simulink library "AEMS_Standard_Library"  (R2016b)
settings: Solver=ode45  StartTime=0.0  StopTime=10.0  RelTol=1e-3
undefined symbols (not defined in the file or in its folder): BkPY, carto, Cbx_extegr, Cbx_lpegrsys, Cbx_portegr, Cnx_bnk_nr_conf, Cnx_cyl_nr_conf, ConfigManagement, configuration_management, Cxx_dcm_io_tmr_end_xxxx, Cxx_dcm_rt_tmr_end, Cxx_DID_xxxx_IO_max, Cxx_DID_xxxx_IO_min, Cxx_egrhsofs, Cxx_vmaniegi, DEM_DEBOUNCE_FREEZE, DEM_DTR_CTL_INVISIBLE, DEM_DTR_CTL_NORMAL, Dem_DtrId2_XXX, Dem_DtrId3_XXX, Dem_DtrId4_XXX, Dem_DtrId5_XXX, Dem_DtrId6_XXX, Dem_DtrId7_XXX, Dem_DtrId8_XXX, Dem_DtrId9_XXX, Dem_DtrId_XXX, Dem_EnableConditionId2_XXX, Dem_EnableConditionId3_XXX, Dem_EnableConditionId4_XXX, Dem_EnableConditionId5_XXX, Dem_EnableConditionId6_XXX, Dem_EnableConditionId7_XXX, Dem_EnableConditionId8_XXX, Dem_EnableConditionId_XXX, Dem_EventId, Dem_EventId2_XXX, Dem_EventId3_XXX, Dem_EventId4_XXX, Dem_EventId5_XXX, Dem_EventId6_XXX, Dem_EventId7_XXX, Dem_EventId8_XXX, Dem_EventId9_XXX, Dem_EventId_Device_Faulttype, Dem_EventId_XXX, DEM_IUMPR_GENERAL_DENOMINATOR, DEM_OPCYC_IGNITION, Dem_RatioId2_XXX, Dem_RatioId3_XXX, Dem_RatioId4_XXX, Dem_RatioId5_XXX, Dem_RatioId6_XXX, Dem_RatioId7_XXX, Dem_RatioId8_XXX, Dem_RatioId_XXX, Dem_StorageConditionId2_XXX, Dem_StorageConditionId3_XXX, Dem_StorageConditionId4_XXX, Dem_StorageConditionId5_XXX ... (+65)
libraries: AEMS_Standard_Library x477, simulink x2
(part 37 of 39)

== system AEMS_Standard_Library/SPECIFIC/AEMS_AIR_BALANCE/MWI_Mani_Charge_Mass_Air_EGR/MWI_egrmani_pm_cal ==
  qcylegr_pudt : Inport  Interpolate=off
  fair_egrv : Inport  Port=2  Interpolate=off
  qegrve : Inport  Port=3  Interpolate=off
  egrmani_cal_ok : EnablePort
      settings: AttributesFormatString=<states=%<StatesWhenEnabling>>
  Product4 : Product  Inputs=*/  SaturateOnIntegerOverflow=on  RndMeth=Zero  InputSameDT=on
  Saturation1 : Saturate  UpperLimit=100  LowerLimit=0
      settings: AttributesFormatString=<limits=%<UpperLimit>/%<LowerLimit>>
  Sum : Sum  Inputs=+-  SaturateOnIntegerOverflow=on  InputSameDT=on
  Sum1 : Sum  SaturateOnIntegerOverflow=on  InputSameDT=on
  Switch : Switch  Criteria=u2 ~= 0  SaturateOnIntegerOverflow=on  InputSameDT=on
      settings: AttributesFormatString=Criteria=%<Criteria>
  Unit Delay3 : UnitDelay  SampleTime=-1
      settings: AttributesFormatString=<initial=%<InitialCondition>>
  g_per_s_to_g_per_freq : Constant  Value=500  OutDataTypeStr=single
  g_per_s_to_g_per_frq : Constant  Value=0  OutDataTypeStr=single
  egrmani : Outport  InitialOutput=0
      settings: AttributesFormatString=<initial=%<InitialOutput>>\n<whendisabled=%<OutputWhenDisabled>>
  wires:
  Product4/1 -> Sum1/2
  Unit Delay3/1 -> Sum1/1
  g_per_s_to_g_per_freq/1 -> Product4/2
  Saturation1/1 -> Unit Delay3/1, egrmani/1  "egrmani"
  Sum1/1 -> Saturation1/1
  Sum/1 -> Product4/1
  qcylegr_pudt/1 -> Sum/2
  qegrve/1 -> Switch/3
  g_per_s_to_g_per_frq/1 -> Switch/1
  fair_egrv/1 -> Switch/2
  Switch/1 -> Sum/1

== system AEMS_Standard_Library/SPECIFIC/AEMS_AIR_BALANCE/MWI_Mani_Charge_Mass_Air_EGR/MWI_mamani_pm_cal ==
  egrmani : Inport  Interpolate=off
  qegrth : Inport  Port=2  Interpolate=off
  fqselgo : Inport  Port=3  Interpolate=off
  pargeqd : Inport  Port=4  Interpolate=off
  tanmnp : Inport  Port=5  Interpolate=off
  ppamb : Inport  Port=6  Interpolate=off
  qtrm : Inport  Port=7  Interpolate=off
  qcyl_pudt : Inport  Port=8  Interpolate=off
  qcylall_pudt : Inport  Port=9  Interpolate=off
  fafmlmsta : Inport  Port=10  Interpolate=off
  vmani : Inport  Port=11  Interpolate=off
  qegrve : Inport  Port=12  Interpolate=off
  fair_egrv : Inport  Port=13  Interpolate=off
  Constant : Constant  Value=0  OutDataTypeStr=single
  Constant1 : Constant  Value=Cbx_lpegrsys
  Constant2 : Constant  Value=100  OutDataTypeStr=single
  MinMax : MinMax  Function=max  Inputs=2  SaturateOnIntegerOverflow=on  InputSameDT=on
  MinMax1 : MinMax  Inputs=2  SaturateOnIntegerOverflow=on  InputSameDT=on
  MinMax2 : MinMax  Function=max  Inputs=2  SaturateOnIntegerOverflow=on  InputSameDT=on
  Product : Product  Inputs=*/  SaturateOnIntegerOverflow=on  RndMeth=Zero  InputSameDT=on
  Product1 : Product  SaturateOnIntegerOverflow=on  RndMeth=Zero  InputSameDT=on
  Product2 : Product  SaturateOnIntegerOverflow=on  RndMeth=Zero  InputSameDT=on
  Product3 : Product  Inputs=*/  SaturateOnIntegerOverflow=on  RndMeth=Zero  InputSameDT=on
  Sum1 : Sum  Inputs=+-  SaturateOnIntegerOverflow=on  InputSameDT=on
  Sum{2..3,5..6} (4 alike) : Sum  SaturateOnIntegerOverflow=on  InputSameDT=on
  Sum4 : Sum  Inputs=+++  SaturateOnIntegerOverflow=on  InputSameDT=on
  Sum7 : Sum  Inputs=+-  SaturateOnIntegerOverflow=on  InputSameDT=on
  Switch{,1..3} (4 alike) : Switch  Criteria=u2 ~= 0  SaturateOnIntegerOverflow=on  InputSameDT=on
      settings: AttributesFormatString=Criteria=%<Criteria>
  Unit Delay1 : UnitDelay  SampleTime=-1
      settings: AttributesFormatString=<initial=%<InitialCondition>>
  constant : Constant  Value=0.00028704  OutDataTypeStr=single
  constant1 : Constant  Value=273  OutDataTypeStr=single
  constant2 : Constant  Value=0.00028704  OutDataTypeStr=single
  g/s_to_g/2ms1 : Constant  Value=500  OutDataTypeStr=single
  g/s_to_g/2ms2 : Constant  Value=0  OutDataTypeStr=single
  mVMANI1 : Constant  Value=Cxx_vmaniegi
  mamani : Outport
  airmani : Outport  Port=2
  wires:
  vmani/1 -> Sum5/2
  MinMax/1 -> Switch/3  "airmani"
  Switch2/1 -> MinMax1/1
  Sum2/1 -> MinMax1/2
  Constant/1 -> MinMax/2
  MinMax1/1 -> MinMax/1
  Constant2/1 -> Switch2/3
  fafmlmsta/1 -> Switch2/2
  pargeqd/1 -> Sum4/2
  qegrth/1 -> Sum7/2
  qcylall_pudt/1 -> Sum7/1
  Sum7/1 -> Switch1/1
  qcyl_pudt/1 -> Switch1/3
  Constant1/1 -> Switch1/2
  Switch1/1 -> Sum1/2
  Sum1/1 -> Product3/1
  constant2/1 -> MinMax2/1
  Product2/1 -> MinMax2/2
  MinMax2/1 -> Product/2
  egrmani/1 -> Sum6/2
  Sum6/1 -> mamani/1  "mamani"
  fqselgo/1 -> Switch/2
  Sum5/1 -> Product1/1
  mVMANI1/1 -> Sum5/1
  Switch/1 -> Sum6/1, Unit Delay1/1, airmani/1  "airmani"
  ppamb/1 -> Product1/2
  Product/1 -> Switch2/1, Switch/1  "mamani_ini"
  constant1/1 -> Sum3/2
  Sum3/1 -> Product2/2
  tanmnp/1 -> Sum3/1
  constant/1 -> Product2/1
  Product1/1 -> Product/1
  g/s_to_g/2ms1/1 -> Product3/2
  Product3/1 -> Sum2/1
  qtrm/1 -> Sum4/1
  Unit Delay1/1 -> Sum2/2
  Switch3/1 -> Sum4/3
  qegrve/1 -> Switch3/1
  g/s_to_g/2ms2/1 -> Switch3/3
  Sum4/1 -> Sum1/1
  fair_egrv/1 -> Switch3/2

== system AEMS_Standard_Library/SPECIFIC/AEMS_AS_PADE/A_pade_model/A_filter_pade ==
  Vxx_in_fil : Inport
  Vxx_dly_t : Inport  Port=2
  Vbx_dly_init_ena : Inport  Port=3
  A_filter_1 : Subsystem
  B_filter_2 : Subsystem
  C_filter_3 : Subsystem
  Vxx_in_dly : Outport
  wires:
  Vxx_dly_t/1 -> A_filter_1/1(Vxx_dly_t), C_filter_3/1(Vxx_dly_t), B_filter_2/1(Vxx_dly_t)
  Vbx_dly_init_ena/1 -> C_filter_3/3(Vbx_dly_init_ena), B_filter_2/3(Vbx_dly_init_ena), A_filter_1/3(Vbx_dly_init_ena)
  C_filter_3/1(Vxx_in_dly) -> Vxx_in_dly/1
  B_filter_2/1(Vxx_dly_2) -> C_filter_3/2(Vxx_dly_2)
  Vxx_in_fil/1 -> C_filter_3/4(Vxx_in_fil), B_filter_2/4(Vxx_in_fil), A_filter_1/2(Vxx_in_fil)
  A_filter_1/1(Vxx_dly_1) -> B_filter_2/2(Vxx_dly_1)

== system AEMS_Standard_Library/SPECIFIC/AEMS_AT_EHR/A_Enabled_Calculation/A_Calcul_for_all_bricks ==
  Vxx_ehr_cnvt_fac : Inport
  Vxx_ehr_ext_exch_ar : Inport  Port=2
  Vxx_ehr_samp_t : Inport  Port=3
  Product1 : Product  OutDataTypeStr=Inherit: Inherit via back propagation  RndMeth=Zero
  Product5 : Product  OutDataTypeStr=Inherit: Inherit via back propagation  RndMeth=Zero
  Vxx_ehr_ext_cnvt_entr : Outport
  wires:
  Product1/1 -> Vxx_ehr_ext_cnvt_entr/1
  Product5/1 -> Product1/1
  Vxx_ehr_samp_t/1 -> Product1/2
  Vxx_ehr_ext_exch_ar/1 -> Product5/2
  Vxx_ehr_cnvt_fac/1 -> Product5/1

== system AEMS_Standard_Library/SPECIFIC/AEMS_AT_EHR/A_Enabled_Calculation/B_Temp_calculation_in_brick ==
  Vxx_ehr_ext_cnvt_entr : Inport
  Vxx_ehr_samp_t : Inport  Port=2
  Vxx_ehr_sel_tenv : Inport  Port=3
  Vxx_ehr_spc_ex_gas_temp_cpy : Inport  Port=4
  Vxx_ehr_spc_cata_temp_cpy : Inport  Port=5
  Vxx_ehr_sys_egaf : Inport  Port=6
  Vxx_ehr_exo_pow : Inport  Port=7
  Vxx_ehr_wht : Inport  Port=8
  Vxx_ehr_utp : Inport  Port=9
  Vxx_ehr_cata_temp_dly : Inport  Port=10
  A_Entropy_calculation : Subsystem
  B_Temp_fluctuation_calculation : Subsystem
  C_Temp_and_power_calculation : Subsystem
  Saturation{,1..3} (4 alike) : Saturate  UpperLimit=1240  LowerLimit=0  RndMeth=Zero
      settings: AttributesFormatString=<limits=%<UpperLimit>/%<LowerLimit>>
  Saturation7 : Saturate  UpperLimit=32767  LowerLimit=-32767  RndMeth=Zero
      settings: AttributesFormatString=<limits=%<UpperLimit>/%<LowerLimit>>
  Vxx_ehr_dtp : Outport
  Vxx_ehr_ext_pow_loss : Outport  Port=2
  Vxx_ehr_wht_entr : Outport  Port=3
  Vxx_ehr_ex_gas_entr : Outport  Port=4
  Vxx_ehr_exo_temp_flu : Outport  Port=5
  Vxx_ehr_wht_temp_flu : Outport  Port=6
  Vxx_ehr_ex_gas_temp_flu : Outport  Port=7
  Vxx_ehr_ext_cnvt_temp_flu : Outport  Port=8
  wires:
  Saturation3/1 -> Vxx_ehr_ext_cnvt_temp_flu/1, C_Temp_and_power_calculation/4(Vxx_ehr_ext_cnvt_temp_flu)
  Saturation2/1 -> C_Temp_and_power_calculation/3(Vxx_ehr_ex_gas_temp_flu), Vxx_ehr_ex_gas_temp_flu/1
  Saturation1/1 -> Vxx_ehr_wht_temp_flu/1, C_Temp_and_power_calculation/2(Vxx_ehr_wht_temp_flu)
  Saturation/1 -> Vxx_ehr_exo_temp_flu/1, C_Temp_and_power_calculation/1(Vxx_ehr_exo_temp_flu)
  Saturation7/1 -> Vxx_ehr_ext_pow_loss/1
  C_Temp_and_power_calculation/1(Vxx_ehr_ext_pow_loss) -> Saturation7/1
  B_Temp_fluctuation_calculation/4(Vxx_ehr_ext_cnvt_temp_flu) -> Saturation3/1
  B_Temp_fluctuation_calculation/3(Vxx_ehr_ex_gas_temp_flu) -> Saturation2/1
  B_Temp_fluctuation_calculation/2(Vxx_ehr_wht_temp_flu) -> Saturation1/1
  B_Temp_fluctuation_calculation/1(Vxx_ehr_exo_temp_flu) -> Saturation/1
  A_Entropy_calculation/6(Vxx_ehr_ext_cnvt_entr_rat) -> B_Temp_fluctuation_calculation/4(Vxx_ehr_ext_cnvt_entr_rat)
  A_Entropy_calculation/5(Vxx_ehr_ex_gas_entr_rat) -> B_Temp_fluctuation_calculation/3(Vxx_ehr_ex_gas_entr_rat)
  C_Temp_and_power_calculation/2(Vxx_ehr_dtp) -> Vxx_ehr_dtp/1
  A_Entropy_calculation/4(Vxx_ehr_wht_entr_rat) -> B_Temp_fluctuation_calculation/2(Vxx_ehr_wht_entr_rat)
  A_Entropy_calculation/3(Vxx_ehr_ex_gas_entr) -> Vxx_ehr_ex_gas_entr/1
  A_Entropy_calculation/1(Vxx_ehr_entr_tot) -> B_Temp_fluctuation_calculation/1(Vxx_ehr_entr_tot)
  A_Entropy_calculation/2(Vxx_ehr_wht_entr) -> Vxx_ehr_wht_entr/1
  Vxx_ehr_wht/1 -> A_Entropy_calculation/4(Vxx_ehr_wht)
  Vxx_ehr_cata_temp_dly/1 -> B_Temp_fluctuation_calculation/8(Vxx_ehr_cata_temp_dly)
  Vxx_ehr_sys_egaf/1 -> A_Entropy_calculation/2(Vxx_ehr_sys_egaf)
  Vxx_ehr_exo_pow/1 -> B_Temp_fluctuation_calculation/6(Vxx_ehr_exo_pow)
  Vxx_ehr_spc_cata_temp_cpy/1 -> A_Entropy_calculation/1(Vxx_ehr_spc_cata_temp_cpy)
  Vxx_ehr_spc_ex_gas_temp_cpy/1 -> A_Entropy_calculation/3(Vxx_ehr_spc_ex_gas_temp_cpy)
  Vxx_ehr_ext_cnvt_entr/1 -> A_Entropy_calculation/5(Vxx_ehr_ext_cnvt_entr), C_Temp_and_power_calculation/7(Vxx_ehr_ext_cnvt_entr)
  Vxx_ehr_utp/1 -> B_Temp_fluctuation_calculation/7(Vxx_ehr_utp)
  Vxx_ehr_samp_t/1 -> A_Entropy_calculation/6(Vxx_ehr_samp_t), B_Temp_fluctuation_calculation/5(Vxx_ehr_samp_t), C_Temp_and_power_calculation/6(Vxx_ehr_samp_t)
  Vxx_ehr_sel_tenv/1 -> B_Temp_fluctuation_calculation/9(Vxx_ehr_sel_tenv), C_Temp_and_power_calculation/5(Vxx_ehr_sel_tenv)

== system AEMS_Standard_Library/SPECIFIC/AEMS_AT_TUBE/A_Thermal_Calculation/A_Thermal_Convection_Terms_Tube ==
  Vxx_tub_itl_cnvt_fac : Inport
  Vxx_tub_itl_ar : Inport  Port=2
  Vxx_tub_ext_cnvt_fac : Inport  Port=3
  Vxx_tub_ext_ar : Inport  Port=4
  hextSext : Product  Inputs=**  OutDataTypeStr=Inherit: Inherit via back propagation  RndMeth=Zero
  hextSext1 : Product  Inputs=**  OutDataTypeStr=Inherit: Inherit via back propagation  RndMeth=Zero
  Vxx_tub_ext_ar_cnvt_fac : Outport
  Vxx_tub_itl_ar_cnvt_fac : Outport  Port=2
  wires:
  Vxx_tub_itl_ar/1 -> hextSext1/2
  Vxx_tub_itl_cnvt_fac/1 -> hextSext1/1
  Vxx_tub_ext_ar/1 -> hextSext/2
  Vxx_tub_ext_cnvt_fac/1 -> hextSext/1
  hextSext1/1 -> Vxx_tub_itl_ar_cnvt_fac/1
  hextSext/1 -> Vxx_tub_ext_ar_cnvt_fac/1

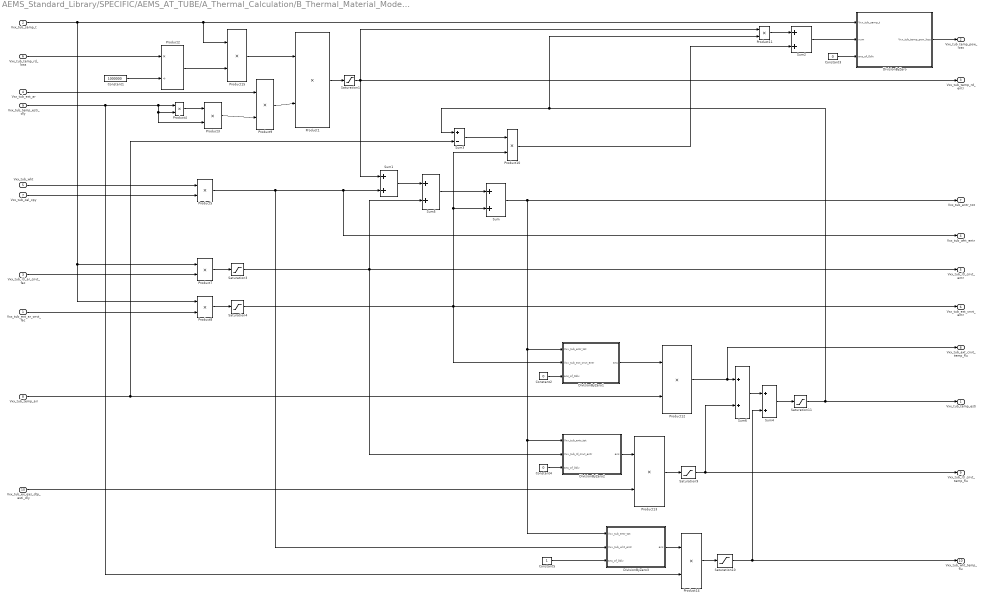
== system AEMS_Standard_Library/SPECIFIC/AEMS_AT_TUBE/A_Thermal_Calculation/B_Thermal_Material_Model_Tube ==
  Vxx_tub_ext_ar_cnvt_fac : Inport
  Vxx_tub_samp_t : Inport  Port=2
  Vxx_tub_itl_ar_cnvt_fac : Inport  Port=3
  Vxx_tub_ext_ar : Inport  Port=4
  Vxx_tub_wht : Inport  Port=5
  Vxx_tub_temp_rd_loss : Inport  Port=6
  Vxx_tub_cal_cpy : Inport  Port=7
  Vxx_tub_temp_air : Inport  Port=8
  Vxx_tub_temp_esti_dly : Inport  Port=9
  Vxx_tub_ex_gas_dtp_esti_dly : Inport  Port=10
  Constant1 : Constant  Value=1000000  OutDataTypeStr=Inherit: Inherit via back propagation
  Constant2 : Constant  Value=0  OutDataTypeStr=Inherit: Inherit via back propagation
  Constant3 : Constant  Value=0  OutDataTypeStr=Inherit: Inherit via back propagation
  Constant4 : Constant  Value=0  OutDataTypeStr=Inherit: Inherit via back propagation
  Constant5 : Constant  OutDataTypeStr=Inherit: Inherit via back propagation
  DivisionByZero : Subsystem
  DivisionByZero1 : Subsystem
  DivisionByZero2 : Subsystem
  DivisionByZero3 : Subsystem
  Product{1,3..4,9,15} (5 alike) : Product  OutDataTypeStr=Inherit: Inherit via back propagation  RndMeth=Zero
  Product{5,7..8,10..14} (8 alike) : Product  Inputs=**  OutDataTypeStr=Inherit: Inherit via back propagation  RndMeth=Zero
  Product2 : Product  Inputs=*/  OutDataTypeStr=Inherit: Inherit via back propagation  RndMeth=Zero
  Saturation1 : Saturate  UpperLimit=6.5535  LowerLimit=0  RndMeth=Zero
      settings: AttributesFormatString=<limits=%<UpperLimit>/%<LowerLimit>>
  Saturation10 : Saturate  UpperLimit=1240  LowerLimit=0  RndMeth=Zero
      settings: AttributesFormatString=<limits=%<UpperLimit>/%<LowerLimit>>
  Saturation11 : Saturate  UpperLimit=1473  LowerLimit=233  RndMeth=Zero
      settings: AttributesFormatString=<limits=%<UpperLimit>/%<LowerLimit>>
  Saturation3 : Saturate  UpperLimit=1310.6  LowerLimit=0  RndMeth=Zero
      settings: AttributesFormatString=<limits=%<UpperLimit>/%<LowerLimit>>
  Saturation4 : Saturate  UpperLimit=6.5535  LowerLimit=0  RndMeth=Zero
      settings: AttributesFormatString=<limits=%<UpperLimit>/%<LowerLimit>>
  Saturation9 : Saturate  UpperLimit=1240  LowerLimit=0  RndMeth=Zero
      settings: AttributesFormatString=<limits=%<UpperLimit>/%<LowerLimit>>
  Sum{,1..2,4..5} (5 alike) : Sum  Inputs=2  OutDataTypeStr=Inherit: Inherit via back propagation  RndMeth=Zero  InputSameDT=on
  Sum3 : Sum  Inputs=+-  OutDataTypeStr=Inherit: Inherit via back propagation  RndMeth=Zero  InputSameDT=on
  Sum6 : Sum  OutDataTypeStr=Inherit: Inherit via back propagation  RndMeth=Zero  InputSameDT=on
  Vxx_tub_temp_esti : Outport
  Vxx_tub_temp_pow_loss : Outport  Port=2
  Vxx_tub_temp_rd_entr : Outport  Port=3
  Vxx_tub_wht_entr : Outport  Port=4
  Vxx_tub_itl_cnvt_entr : Outport  Port=5
  Vxx_tub_ext_cnvt_entr : Outport  Port=6
  Vxx_tub_entr_tot : Outport  Port=7
  Vxx_tub_ext_cnvt_temp_flu : Outport  Port=8
  Vxx_tub_itl_cnvt_temp_flu : Outport  Port=9
  Vxx_tub_wht_temp_flu : Outport  Port=10
  wires:
  Saturation11/1 -> Vxx_tub_temp_esti/1, Product11/2, Sum3/1
  DivisionByZero/1(Vxx_tub_temp_pow_loss) -> Vxx_tub_temp_pow_loss/1
  Constant3/1 -> DivisionByZero/3(ans_of_0div)
  Sum2/1 -> DivisionByZero/2(num)
  Saturation9/1 -> Sum6/2, Vxx_tub_itl_cnvt_temp_flu/1
  Saturation10/1 -> Sum4/2, Vxx_tub_wht_temp_flu/1
  Saturation4/1 -> Vxx_tub_ext_cnvt_entr/1, Product10/2, Sum/2, DivisionByZero1/2(Vxx_tub_ext_cnvt_entr)
  Saturation3/1 -> DivisionByZero2/2(Vxx_tub_itl_cnvt_entr), Sum5/2, Vxx_tub_itl_cnvt_entr/1
  Saturation1/1 -> Sum1/1, Vxx_tub_temp_rd_entr/1, Product11/1
  Product9/1 -> Product1/2
  Product15/1 -> Product1/1
  Vxx_tub_ext_ar/1 -> Product9/1
  Product3/1 -> Product9/2
  Constant5/1 -> DivisionByZero3/3(ans_of_0div)
  Constant4/1 -> DivisionByZero2/3(ans_of_0div)
  Constant2/1 -> DivisionByZero1/3(ans_of_0div)
  Vxx_tub_temp_esti_dly/1 -> Product3/2, Product4/2, Product4/1, Product14/2
  Sum3/1 -> Product10/1
  Product10/1 -> Sum2/2
  Product11/1 -> Sum2/1
  Vxx_tub_temp_air/1 -> Sum3/2, Product12/2
  Vxx_tub_itl_ar_cnvt_fac/1 -> Product7/2
  Constant1/1 -> Product2/2
  Vxx_tub_temp_rd_loss/1 -> Product2/1
  Vxx_tub_cal_cpy/1 -> Product5/2
  Vxx_tub_wht/1 -> Product5/1
  Vxx_tub_ext_ar_cnvt_fac/1 -> Product8/2
  Product8/1 -> Saturation4/1
  DivisionByZero1/1(ans) -> Product12/1
  Product12/1 -> Sum6/1, Vxx_tub_ext_cnvt_temp_flu/1
  Product7/1 -> Saturation3/1
  Product13/1 -> Saturation9/1
  Product1/1 -> Saturation1/1
  Product5/1 -> DivisionByZero3/2(Vxx_tub_wht_entr), Vxx_tub_wht_entr/1, Sum1/2
  DivisionByZero3/1(ans) -> Product14/1
  Product14/1 -> Saturation10/1
  Sum4/1 -> Saturation11/1
  DivisionByZero2/1(ans) -> Product13/1
  Vxx_tub_ex_gas_dtp_esti_dly/1 -> Product13/2
  Product4/1 -> Product3/1
  Sum/1 -> DivisionByZero1/1(Vxx_tub_entr_tot), DivisionByZero2/1(Vxx_tub_entr_tot), DivisionByZero3/1(Vxx_tub_entr_tot), Vxx_tub_entr_tot/1
  Sum1/1 -> Sum5/1
  Sum5/1 -> Sum/1
  Sum6/1 -> Sum4/1
  Vxx_tub_samp_t/1 -> Product8/1, Product7/1, Product15/1, DivisionByZero/1(Vxx_tub_samp_t)
  Product2/1 -> Product15/2

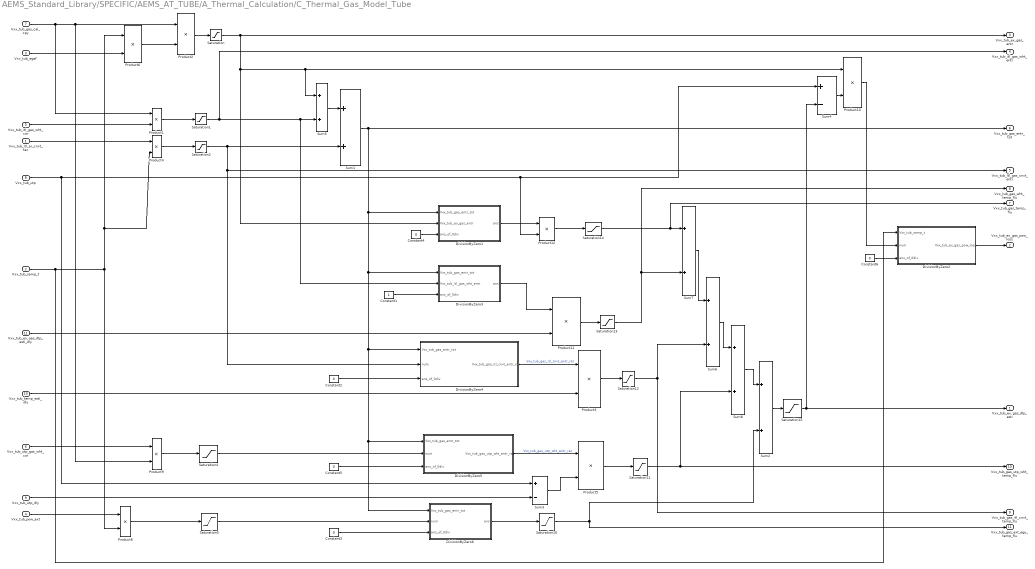
== system AEMS_Standard_Library/SPECIFIC/AEMS_AT_TUBE/A_Thermal_Calculation/C_Thermal_Gas_Model_Tube ==
  Vxx_tub_itl_ar_cnvt_fac : Inport
  Vxx_tub_samp_t : Inport  Port=2
  Vxx_tub_egaf : Inport  Port=3
  Vxx_tub_pow_ext : Inport  Port=4
  Vxx_tub_itl_gas_wht_cor : Inport  Port=5
  Vxx_tub_utp_gas_wht_cor : Inport  Port=6
  Vxx_tub_gas_cal_cpy : Inport  Port=7
  Vxx_tub_utp : Inport  Port=8
  Vxx_tub_utp_dly : Inport  Port=9
  Vxx_tub_temp_esti_dly : Inport  Port=10
  Vxx_tub_ex_gas_dtp_esti_dly : Inport  Port=11  PortDimensions=1
  Constant1 : Constant  OutDataTypeStr=Inherit: Inherit via back propagation
  Constant{2..6} (5 alike) : Constant  Value=0  OutDataTypeStr=Inherit: Inherit via back propagation
  DivisionByZero1 : Subsystem
  DivisionByZero2 : Subsystem
  DivisionByZero3 : Subsystem
  DivisionByZero4 : Subsystem
  DivisionByZero5 : Subsystem
  DivisionByZero6 : Subsystem
  Product{1..6,8..12} (11 alike) : Product  OutDataTypeStr=Inherit: Inherit via back propagation  RndMeth=Zero
  Saturation : Saturate  UpperLimit=65.535  LowerLimit=0  RndMeth=Zero
      settings: AttributesFormatString=<limits=%<UpperLimit>/%<LowerLimit>>
  Saturation1 : Saturate  UpperLimit=6553.5  LowerLimit=0  RndMeth=Zero
      settings: AttributesFormatString=<limits=%<UpperLimit>/%<LowerLimit>>
  Saturation10 : Saturate  UpperLimit=620  LowerLimit=-620  RndMeth=Zero
      settings: AttributesFormatString=<limits=%<UpperLimit>/%<LowerLimit>>
  Saturation11 : Saturate  UpperLimit=620  LowerLimit=-620  RndMeth=Zero
      settings: AttributesFormatString=<limits=%<UpperLimit>/%<LowerLimit>>
  Saturation12 : Saturate  UpperLimit=1240  LowerLimit=0  RndMeth=Zero
      settings: AttributesFormatString=<limits=%<UpperLimit>/%<LowerLimit>>
  Saturation13 : Saturate  UpperLimit=1240  LowerLimit=0  RndMeth=Zero
      settings: AttributesFormatString=<limits=%<UpperLimit>/%<LowerLimit>>
  Saturation14 : Saturate  UpperLimit=1240  LowerLimit=0  RndMeth=Zero
      settings: AttributesFormatString=<limits=%<UpperLimit>/%<LowerLimit>>
  Saturation15 : Saturate  UpperLimit=1473  LowerLimit=233  RndMeth=Zero
      settings: AttributesFormatString=<limits=%<UpperLimit>/%<LowerLimit>>
  Saturation2 : Saturate  UpperLimit=1310.6  LowerLimit=0  RndMeth=Zero
      settings: AttributesFormatString=<limits=%<UpperLimit>/%<LowerLimit>>
  Saturation4 : Saturate  UpperLimit=3276.7  LowerLimit=-3276.6  RndMeth=Zero
      settings: AttributesFormatString=<limits=%<UpperLimit>/%<LowerLimit>>
  Saturation5 : Saturate  UpperLimit=32767  LowerLimit=-32767  RndMeth=Zero
      settings: AttributesFormatString=<limits=%<UpperLimit>/%<LowerLimit>>
  Sum1 : Sum  Inputs=2  OutDataTypeStr=Inherit: Inherit via back propagation  RndMeth=Zero  InputSameDT=on
  Sum{2,6..8} (4 alike) : Sum  OutDataTypeStr=Inherit: Inherit via back propagation  RndMeth=Zero  InputSameDT=on
  Sum3 : Sum  Inputs=+-  OutDataTypeStr=Inherit: Inherit via back propagation  RndMeth=Zero  InputSameDT=on
  Sum4 : Sum  Inputs=+-  OutDataTypeStr=Inherit: Inherit via back propagation  RndMeth=Zero  InputSameDT=on
  Sum5 : Sum  Inputs=2  OutDataTypeStr=Inherit: Inherit via back propagation  RndMeth=Zero  InputSameDT=on
  Vxx_tub_ex_gas_dtp_esti : Outport
  Vxx_tub_ex_gas_pow_loss : Outport  Port=2
  Vxx_tub_ex_gas_entr : Outport  Port=3
  Vxx_tub_itl_gas_wht_entr : Outport  Port=4
  Vxx_tub_itl_gas_cnvt_entr : Outport  Port=5
  Vxx_tub_gas_entr_tot : Outport  Port=6
  Vxx_tub_gas_temp_flu : Outport  Port=7
  Vxx_tub_gas_wht_temp_flu : Outport  Port=8
  Vxx_tub_gas_itl_cnvt_temp_flu : Outport  Port=9
  Vxx_tub_gas_utp_wht_temp_flu : Outport  Port=10
  Vxx_tub_gas_ext_egy_temp_flu : Outport  Port=11
  wires:
  Sum1/1 -> DivisionByZero6/1(Vxx_tub_gas_entr_tot), DivisionByZero5/1(Vxx_tub_gas_entr_tot), DivisionByZero4/1(Vxx_tub_gas_entr_tot), DivisionByZero3/1(Vxx_tub_gas_entr_tot), DivisionByZero1/1(Vxx_tub_gas_entr_tot), Vxx_tub_gas_entr_tot/1
  Saturation4/1 -> DivisionByZero5/2(num)
  Saturation5/1 -> DivisionByZero6/2(num)
  Saturation14/1 -> Sum7/1, Vxx_tub_gas_temp_flu/1
  DivisionByZero2/1(Vxx_tub_ex_gas_pow_loss) -> Vxx_tub_ex_gas_pow_loss/1
  Product10/1 -> DivisionByZero2/2(num)
  Constant6/1 -> DivisionByZero2/3(ans_of_0div)
  Saturation15/1 -> Vxx_tub_ex_gas_dtp_esti/1, Sum4/2
  Saturation11/1 -> Sum8/2, Vxx_tub_gas_utp_wht_temp_flu/1
  Saturation12/1 -> Sum6/2, Vxx_tub_gas_itl_cnvt_temp_flu/1
  Saturation13/1 -> Sum7/2, Vxx_tub_gas_wht_temp_flu/1
  Saturation10/1 -> Sum2/2, Vxx_tub_gas_ext_egy_temp_flu/1
  Saturation2/1 -> DivisionByZero4/2(num), Vxx_tub_itl_gas_cnvt_entr/1, Sum1/2
  Saturation1/1 -> DivisionByZero3/2(Vxx_tub_itl_gas_wht_entr), Sum5/2, Vxx_tub_itl_gas_wht_entr/1
  Saturation/1 -> Vxx_tub_ex_gas_entr/1, DivisionByZero1/2(Vxx_tub_ex_gas_entr), Sum5/1, Product10/1
  Sum4/1 -> Product10/2
  Vxx_tub_utp_dly/1 -> Sum3/2
  Sum3/1 -> Product5/2
  Vxx_tub_pow_ext/1 -> Product8/1
  Vxx_tub_itl_ar_cnvt_fac/1 -> Product4/1
  Vxx_tub_temp_esti_dly/1 -> Product3/2
  Vxx_tub_ex_gas_dtp_esti_dly/1 -> Product11/2
  Constant5/1 -> DivisionByZero5/3(ans_of_0div)
  Constant4/1 -> DivisionByZero1/3(ans_of_0div)
  Constant3/1 -> DivisionByZero6/3(ans_of_0div)
  Constant2/1 -> DivisionByZero4/3(ans_of_0div)
  Constant1/1 -> DivisionByZero3/3(ans_of_0div)
  Vxx_tub_utp_gas_wht_cor/1 -> Product9/1
  Vxx_tub_itl_gas_wht_cor/1 -> Product1/2
  Vxx_tub_egaf/1 -> Product6/2
  Product2/1 -> Saturation/1
  Product8/1 -> Saturation5/1
  DivisionByZero1/1(ans) -> Product12/1
  DivisionByZero6/1(ans) -> Saturation10/1
  DivisionByZero4/1(Vxx_tub_gas_itl_cnvt_entr_rat) -> Product3/1  "Vxx_tub_gas_itl_cnvt_entr_rat"
  Product3/1 -> Saturation12/1
  Product12/1 -> Saturation14/1
  DivisionByZero5/1(Vxx_tub_gas_utp_wht_entr_rat) -> Product5/1  "Vxx_tub_gas_utp_wht_entr_rat"
  Product5/1 -> Saturation11/1
  DivisionByZero3/1(ans) -> Product11/1
  Product11/1 -> Saturation13/1
  Product4/1 -> Saturation2/1
  Product1/1 -> Saturation1/1
  Product9/1 -> Saturation4/1
  Sum2/1 -> Saturation15/1
  Sum5/1 -> Sum1/1
  Sum6/1 -> Sum8/1
  Sum7/1 -> Sum6/1
  Sum8/1 -> Sum2/1
  Vxx_tub_gas_cal_cpy/1 -> Product9/2, Product2/1, Product1/1
  Vxx_tub_utp/1 -> Sum4/1, Product12/2, Sum3/1
  Vxx_tub_samp_t/1 -> DivisionByZero2/1(Vxx_tub_samp_t), Product4/2, Product6/1, Product8/2
  Product6/1 -> Product2/2

== system AEMS_Standard_Library/SPECIFIC/AEMS_MULTIPORT_TIMESWITCH_CONFIG/slop_on/SR_FlipFlop ==
  S : Inport
  R : Inport  Port=2
  Constant3 : Constant  Value=true
  Constant5 : Constant  Value=false
  Logical_Operator : Logic  OutDataTypeStr=boolean
  Logical_Operator3 : Logic  Operator=NOT  OutDataTypeStr=boolean
  Switch1 : Switch  Criteria=u2 ~= 0  RndMeth=Zero  InputSameDT=on
      settings: AttributesFormatString=Criteria=%<Criteria>
  Switch2 : Switch  Criteria=u2 ~= 0  RndMeth=Zero  InputSameDT=on
      settings: AttributesFormatString=Criteria=%<Criteria>
  Switch3 : Switch  Criteria=u2 ~= 0  RndMeth=Zero  InputSameDT=on
      settings: AttributesFormatString=Criteria=%<Criteria>
  Unit_Delay : UnitDelay  InitialCondition=initial_condition  SampleTime=-1
      settings: AttributesFormatString=<initial=%<InitialCondition>>
  Q : Outport
  QNot : Outport  Port=2
  wires:
  Logical_Operator3/1 -> QNot/1
  Switch1/1 -> Q/1, Unit_Delay/1, Logical_Operator3/1
  Switch2/1 -> Switch1/3
  Switch3/1 -> Switch2/3
  Constant5/1 -> Switch3/1
  Constant3/1 -> Switch2/1
  Unit_Delay/1 -> Switch3/3, Switch1/1
  S/1 -> Logical_Operator/1, Switch2/2
  R/1 -> Logical_Operator/2, Switch3/2
  Logical_Operator/1 -> Switch1/2

== system AEMS_Standard_Library/SPECIFIC/AEMS_MULTIPORT_TIMESWITCH_CONFIG/transient_timer/DivisionByZero ==
  den : Inport
  num : Inport  Port=2
  ans_of_0div : Inport  Port=3
  Divide : Product  Inputs=*/  OutDataTypeStr=Inherit: Inherit via back propagation  RndMeth=Zero
  MinMax1 : MinMax  Function=max  Inputs=2  OutDataTypeStr=Inherit: Inherit via back propagation  RndMeth=Zero  InputSameDT=on
  RelationalOperator : RelationalOperator  Operator=~=  OutDataTypeStr=boolean  RndMeth=Nearest  InputSameDT=on
  Switch1 : Switch  Criteria=u2 ~= 0  RndMeth=Zero  SaturateOnIntegerOverflow=on  InputSameDT=on
      settings: AttributesFormatString=Criteria=%<Criteria>
  imm_zero : Constant  Value=0  OutDataTypeStr=Inherit: Inherit via back propagation
  imm_zero3 : Constant  Value=1.1920929e-07  OutDataTypeStr=Inherit: Inherit via back propagation
  ans : Outport
  wires:
  imm_zero3/1 -> MinMax1/2
  MinMax1/1 -> Divide/2
  den/1 -> MinMax1/1, RelationalOperator/1
  ans_of_0div/1 -> Switch1/3
  Divide/1 -> Switch1/1
  num/1 -> Divide/1
  Switch1/1 -> ans/1
  imm_zero/1 -> RelationalOperator/2
  RelationalOperator/1 -> Switch1/2

== system AEMS_Standard_Library/SPECIFIC/AEMS_MULTIPORT_TIMESWITCH_CONFIG/transient_timer/UnitDelayResettable ==
  u : Inport
  R : Inport  Port=2
  FixPt_Constant : Constant  DisableCoverage=on  Value=true
  FixPt_Logical_Operator : Logic  DisableCoverage=on  Operator=OR  OutDataTypeStr=boolean
  FixPt_Logical_Operator1 : Logic  DisableCoverage=on  Operator=NOT  OutDataTypeStr=boolean
  FixPt_Unit_Delay1 : UnitDelay  DisableCoverage=on  SampleTime=-1
      settings: AttributesFormatString=<initial=%<InitialCondition>>
  FixPt_Unit_Delay2 : UnitDelay  DisableCoverage=on  InitialCondition=false  SampleTime=-1
      settings: AttributesFormatString=<initial=%<InitialCondition>>
  Init : Switch  Criteria=u2 ~= 0  RndMeth=Zero  ZeroCross=off  InputSameDT=on
      settings: AttributesFormatString=Criteria=%<Criteria>
  Initial_Condition : Constant  DisableCoverage=on  Value=0  OutDataTypeStr=Inherit: Inherit via back propagation
  Reset : Switch  Criteria=u2 ~= 0  RndMeth=Zero  ZeroCross=off  InputSameDT=on
      settings: AttributesFormatString=Criteria=%<Criteria>
  y : Outport
  wires:
  u/1 -> Reset/3
  Initial_Condition/1 -> Reset/1, Init/1  "Initial_Value"
  R/1 -> Reset/2, FixPt_Logical_Operator/1
  FixPt_Logical_Operator/1 -> Init/2
  FixPt_Constant/1 -> FixPt_Unit_Delay2/1
  FixPt_Logical_Operator1/1 -> FixPt_Logical_Operator/2
  Reset/1 -> FixPt_Unit_Delay1/1  "Xnew"
  FixPt_Unit_Delay1/1 -> Init/3  "Xold"
  Init/1 -> y/1
  FixPt_Unit_Delay2/1 -> FixPt_Logical_Operator1/1

== system AEMS_Standard_Library/SPECIFIC/AEMS_SlopeSwitchExtern/Slope_On_Block/Error_Due_To_High_Slope_Test ==
  Signal_Change : Inport
  Output_Less_Than_Input : Inport  Port=2
  Output_Greater_Than_Input : Inport  Port=3
  Logical_Operator1 : Logic  Operator=OR  OutDataTypeStr=boolean
  Relational_Operator3 : RelationalOperator  Operator=~=  OutDataTypeStr=boolean  RndMeth=Nearest  InputSameDT=on
  Unit_Delay1 : UnitDelay  InitialCondition=false  SampleTime=-1
      settings: AttributesFormatString=<initial=%<InitialCondition>>
  Test_passed : Outport
  wires:
  Logical_Operator1/1 -> Test_passed/1
  Signal_Change/1 -> Logical_Operator1/1
  Output_Less_Than_Input/1 -> Unit_Delay1/1
  Output_Greater_Than_Input/1 -> Relational_Operator3/1
  Relational_Operator3/1 -> Logical_Operator1/2
  Unit_Delay1/1 -> Relational_Operator3/2

== system AEMS_Standard_Library/SPECIFIC/AEMS_SlopeSwitchExtern/Slope_On_Block/Output_Comparision ==
  Test_passed : Inport
  Input : Inport  Port=2
  Pos_Slope : Inport  Port=3
  Prev_Output : Inport  Port=4
  Neg_Slope : Inport  Port=5
  Logical_Operator : Logic  Operator=OR  OutDataTypeStr=boolean
  Logical_Operator2 : Logic  OutDataTypeStr=boolean
  Relational_Operator1 : RelationalOperator  Operator=>  OutDataTypeStr=boolean  RndMeth=Nearest  InputSameDT=on
  Relational_Operator2 : RelationalOperator  Operator=<  OutDataTypeStr=boolean  RndMeth=Nearest  InputSameDT=on
  Sum : Sum  OutDataTypeStr=Inherit: Inherit via back propagation  RndMeth=Zero  InputSameDT=on
  Sum1 : Sum  OutDataTypeStr=Inherit: Inherit via back propagation  RndMeth=Zero  InputSameDT=on
  Switch1 : Switch  Criteria=u2 ~= 0  RndMeth=Zero  SaturateOnIntegerOverflow=on  InputSameDT=on
      settings: AttributesFormatString=Criteria=%<Criteria>
  Switch2 : Switch  Criteria=u2 ~= 0  RndMeth=Zero  SaturateOnIntegerOverflow=on  InputSameDT=on
      settings: AttributesFormatString=Criteria=%<Criteria>
  Switch3 : Switch  Criteria=u2 ~= 0  RndMeth=Zero  SaturateOnIntegerOverflow=on  InputSameDT=on
      settings: AttributesFormatString=Criteria=%<Criteria>
  Output_Not_Equals_Input : Outport
  Output : Outport  Port=2
  Output_Less_Than_Input : Outport  Port=3
  Output_Greater_Than_Input : Outport  Port=4
  wires:
  Relational_Operator2/1 -> Output_Less_Than_Input/1, Logical_Operator/1, Switch2/2
  Input/1 -> Relational_Operator2/2, Relational_Operator1/2, Switch1/3, Switch3/3
  Switch2/1 -> Switch3/1
  Switch1/1 -> Switch2/3
  Sum/1 -> Relational_Operator1/1, Switch1/1
  Logical_Operator2/1 -> Output_Not_Equals_Input/1
  Logical_Operator/1 -> Logical_Operator2/2
  Switch3/1 -> Output/1
  Test_passed/1 -> Logical_Operator2/1, Switch3/2
  Relational_Operator1/1 -> Logical_Operator/2, Output_Greater_Than_Input/1, Switch1/2
  Sum1/1 -> Relational_Operator2/1, Switch2/1
  Pos_Slope/1 -> Sum1/1
  Prev_Output/1 -> Sum1/2, Sum/1
  Neg_Slope/1 -> Sum/2

== system AEMS_Standard_Library/COM/AEMS_FRAME_SUPERVISION/ecu_frm_monitoring/B_Status_Management/C_Status_building ==
  Mon_Authorize : Inport
  TimeSched_dt : Inport  Port=2
  JT1 : Inport  Port=3
  JT2 : Inport  Port=4
  Frame_Received : Inport  Port=5
  Status_PREV : Inport  Port=6
  AEMS_UNITDELAY_EXTERNALIC : AEMS_Standard_Library/DISCRETE/AEMS_UNITDELAY_EXTERNALIC  Tag=[LIB]
      settings: AttributesFormatString=%<MaskType>
  Constant2 : Constant  Value=-1  OutDataTypeStr=Inherit: Inherit via back propagation
  Constant4 : Constant  Value=0  OutDataTypeStr=Inherit: Inherit via back propagation
  Constant5 : Constant  Value=false
  DataTypeConversion2 : DataTypeConversion  RndMeth=Zero
  LogicalOperator1 : Logic  Operator=OR  OutDataTypeStr=boolean
  LogicalOperator2 : Logic  Inputs=3  OutDataTypeStr=boolean
  LogicalOperator4 : Logic  Operator=NOT  OutDataTypeStr=boolean
  LogicalOperator5 : Logic  OutDataTypeStr=boolean
  Nsx_abst : Constant  Value=Nnx_abst_stt
  Nsx_pres : Constant  Value=Nnx_pres_stt
  Nsx_vld_abst : Constant  Value=Nnx_vld_abst_stt
  Product : Product  OutDataTypeStr=Inherit: Inherit via back propagation  RndMeth=Zero
  RelationalOperator1 : RelationalOperator  OutDataTypeStr=boolean  RndMeth=Nearest  InputSameDT=on
  RelationalOperator2 : RelationalOperator  OutDataTypeStr=boolean  RndMeth=Nearest  InputSameDT=on
  RelationalOperator3 : RelationalOperator  OutDataTypeStr=boolean  RndMeth=Nearest  InputSameDT=on
  RelationalOperator4 : RelationalOperator  Operator=~=  OutDataTypeStr=boolean  RndMeth=Nearest  InputSameDT=on
  Sum1 : Sum  OutDataTypeStr=Inherit: Inherit via back propagation  RndMeth=Zero  InputSameDT=on
  Sum2 : Sum  Inputs=+-  OutDataTypeStr=Inherit: Inherit via back propagation  RndMeth=Zero  InputSameDT=on
  Switch{1..6} (6 alike) : Switch  Criteria=u2 ~= 0  RndMeth=Zero  InputSameDT=on
      settings: AttributesFormatString=Criteria=%<Criteria>
  UnitDelay2 : UnitDelay  InitialCondition=true  SampleTime=-1
      settings: AttributesFormatString=<initial=%<InitialCondition>>
  UnitDelay3 : UnitDelay  InitialCondition=true  SampleTime=-1
      settings: AttributesFormatString=<initial=%<InitialCondition>>
  Status : Outport
      settings: AttributesFormatString=%<SignalName>
  wires:
  Switch1/1 -> RelationalOperator2/1, RelationalOperator3/1, AEMS_UNITDELAY_EXTERNALIC/1
  Switch4/1 -> Switch6/3
  Sum2/1 -> RelationalOperator1/2
  AEMS_UNITDELAY_EXTERNALIC/1 -> RelationalOperator1/1, Sum1/2
  RelationalOperator1/1 -> Switch3/2
  Sum1/1 -> Switch3/3
  Constant4/1 -> Switch1/1
  Switch3/1 -> Switch1/3
  JT2/1 -> RelationalOperator2/2, Switch3/1, Sum2/1
  RelationalOperator2/1 -> LogicalOperator5/1
  JT1/1 -> RelationalOperator3/2
  Switch2/1 -> Switch4/3
  Nsx_pres/1 -> RelationalOperator4/2, Switch4/1
  Constant5/1 -> UnitDelay2/1
  Mon_Authorize/1 -> LogicalOperator2/2, UnitDelay3/1, LogicalOperator5/2
  LogicalOperator1/1 -> Switch1/2
  UnitDelay3/1 -> LogicalOperator4/1
  LogicalOperator4/1 -> LogicalOperator2/1
  LogicalOperator2/1 -> LogicalOperator1/1
  RelationalOperator4/1 -> LogicalOperator2/3
  DataTypeConversion2/1 -> Status/1
  TimeSched_dt/1 -> Product/1, Sum1/1, Sum2/2
  Constant2/1 -> Product/2
  Product/1 -> AEMS_UNITDELAY_EXTERNALIC/2
  Switch5/1 -> Switch2/3
  Switch6/1 -> DataTypeConversion2/1
  Status_PREV/1 -> Switch6/1, Switch5/3, RelationalOperator4/1
  Frame_Received/1 -> Switch4/2, LogicalOperator1/2
  LogicalOperator5/1 -> Switch2/2
  RelationalOperator3/1 -> Switch5/2
  UnitDelay2/1 -> Switch6/2
  Nsx_abst/1 -> Switch5/1
  Nsx_vld_abst/1 -> Switch2/1

== system AEMS_Standard_Library/MATH/AEMS_SORT/For_loop_1/For_loop_2/Comparison ==
  Vector : Inport
  Index_vector : Inport  Port=2
  Add : Sum
  Constant : Constant  OutDataTypeStr=int8
  Relational_Operator : RelationalOperator  Operator=>  OutDataTypeStr=boolean  RndMeth=Simplest  InputSameDT=on
  Selector : Selector  IndexMode=Zero-based  InputPortWidth=N  IndexOptions=Index vector (port)  Indices=[1 3]  OutputSizes=1
  Selector1 : Selector  IndexMode=Zero-based  InputPortWidth=N  IndexOptions=Index vector (port)  Indices=[1 3]  OutputSizes=1
  Relational_Operator_Boolean : Outport
  High_value_Out : Outport  Port=2
  Low_value_Out : Outport  Port=3
  Low_index_Out : Outport  Port=4
  wires:
  Vector/1 -> Selector/1, Selector1/1
  Index_vector/1 -> Add/1, Selector/2
  Constant/1 -> Add/2
  Selector1/1 -> Low_value_Out/1, Relational_Operator/2
  Add/1 -> Low_index_Out/1, Selector1/2
  Selector/1 -> High_value_Out/1, Relational_Operator/1
  Relational_Operator/1 -> Relational_Operator_Boolean/1

== system AEMS_Standard_Library/MATH/AEMS_SORT/For_loop_1/For_loop_2/Permutation_false ==
  Vector : Inport
  Action Port : ActionPort
  Non_permuted_vector : Outport
  wires:
  Vector/1 -> Non_permuted_vector/1

== system AEMS_Standard_Library/MATH/AEMS_SORT/For_loop_1/For_loop_2/Permutation_true ==
  High_value : Inport
  Low_value : Inport  Port=2
  Low_index : Inport  Port=3
  High_index : Inport  Port=4
  Vector : Inport  Port=5
  Action Port : ActionPort
  Assignment : Assignment  IndexMode=Zero-based  DiagnosticForDimensions=Warning  IndexOptions=Index vector (port)  Indices=1  OutputSizes=1
  Mux : Mux  Inputs=2
  Mux2 : Mux  Inputs=2
  Permuted_vector : Outport
  wires:
  Vector/1 -> Assignment/1
  Mux/1 -> Assignment/2
  Low_value/1 -> Mux/2
  Mux2/1 -> Assignment/3
  Assignment/1 -> Permuted_vector/1
  High_value/1 -> Mux/1
  Low_index/1 -> Mux2/1
  High_index/1 -> Mux2/2

== system AEMS_Standard_Library/MATH/AEMS_SORT/For_loop_1/For_loop_2/Unit_delay_vector ==
  Previous_vector : Inport
  Vector_to_sort : Inport  Port=2
  Index_vector : Inport  Port=3
  Constant1 : Constant  Value=0  OutDataTypeStr=int8
  Logical Operator : Logic  OutDataTypeStr=boolean
  RelationalOperator1 : RelationalOperator  Operator===  OutDataTypeStr=boolean  RndMeth=Nearest  InputSameDT=on
  Switch : Switch  Criteria=u2 ~= 0  RndMeth=Zero  SaturateOnIntegerOverflow=on
      settings: AttributesFormatString=Criteria=%<Criteria>
  UnitDelay1 : UnitDelay  InitialCondition=true  SampleTime=-1
      settings: AttributesFormatString=<initial=%<InitialCondition>>
  Vector_being_sorted : Outport
  wires:
  Logical Operator/1 -> Switch/2
  UnitDelay1/1 -> Logical Operator/2
  RelationalOperator1/1 -> Logical Operator/1, UnitDelay1/1
  Index_vector/1 -> RelationalOperator1/1
  Constant1/1 -> RelationalOperator1/2
  Previous_vector/1 -> Switch/3
  Switch/1 -> Vector_being_sorted/1
  Vector_to_sort/1 -> Switch/1

== system AEMS_Standard_Library/SPECIFIC/AEMS_AS_PADE/A_pade_model/A_filter_pade/A_filter_1 ==
  Vxx_dly_t : Inport
  Vxx_in_fil : Inport  Port=2
  Vbx_dly_init_ena : Inport  Port=3
  AEMS_LUT_1D : AEMS_Standard_Library/LOOKUP_TABLES/AEMS_LUT_1D  Tag=[LIB]  map_x=Cxb_lb_dly_t_para  map_z=Cxp_lb_b0_1
      settings: AttributesFormatString=%<MaskType>\nBkPX=%<map_x>\nLUT=%<map_z>
  AEMS_LUT_1D1 : AEMS_Standard_Library/LOOKUP_TABLES/AEMS_LUT_1D  Tag=[LIB]  map_x=Cxb_lb_dly_t_para  map_z=Cxp_lb_b1_1
      settings: AttributesFormatString=%<MaskType>\nBkPX=%<map_x>\nLUT=%<map_z>
  AEMS_LUT_1D2 : AEMS_Standard_Library/LOOKUP_TABLES/AEMS_LUT_1D  Tag=[LIB]  map_x=Cxb_lb_dly_t_para  map_z=Cxp_lb_a1_1
      settings: AttributesFormatString=%<MaskType>\nBkPX=%<map_x>\nLUT=%<map_z>
  AEMS_LUT_1D3 : AEMS_Standard_Library/LOOKUP_TABLES/AEMS_LUT_1D  Tag=[LIB]  map_x=Cxb_lb_dly_t_para  map_z=Cxp_lb_a2_1
      settings: AttributesFormatString=%<MaskType>\nBkPX=%<map_x>\nLUT=%<map_z>
  A_pade_2nd_order_filter_1 : Subsystem
  Constant1 : Constant  OutDataTypeStr=Inherit: Inherit via back propagation
  Saturation : Saturate  UpperLimit=2000  LowerLimit=0  RndMeth=Zero
      settings: AttributesFormatString=<limits=%<UpperLimit>/%<LowerLimit>>
  Sum1 : Sum  OutDataTypeStr=Inherit: Inherit via back propagation  RndMeth=Zero  InputSameDT=on
  Sum2 : Sum  OutDataTypeStr=Inherit: Inherit via back propagation  RndMeth=Zero  InputSameDT=on
  Sum3 : Sum  Inputs=+-  OutDataTypeStr=Inherit: Inherit via back propagation  RndMeth=Zero  InputSameDT=on
  Sum4 : Sum  Inputs=+-  OutDataTypeStr=Inherit: Inherit via back propagation  RndMeth=Zero  InputSameDT=on
  Vxx_dly_1 : Outport
  wires:
  AEMS_LUT_1D3/1 -> A_pade_2nd_order_filter_1/5(Vxx_a2_1), Sum2/2
  AEMS_LUT_1D2/1 -> A_pade_2nd_order_filter_1/4(Vxx_a1_1), Sum1/2
  AEMS_LUT_1D1/1 -> A_pade_2nd_order_filter_1/2(Vxx_b1_1), Sum3/2
  AEMS_LUT_1D/1 -> A_pade_2nd_order_filter_1/1(Vxx_b0_1), Sum4/2
  Vbx_dly_init_ena/1 -> A_pade_2nd_order_filter_1/7(Vbx_dly_init_ena)
  A_pade_2nd_order_filter_1/1(Vxx_dly_1) -> Saturation/1
  Vxx_in_fil/1 -> A_pade_2nd_order_filter_1/6(Vxx_in_fil)
  Vxx_dly_t/1 -> AEMS_LUT_1D/1, AEMS_LUT_1D1/1, AEMS_LUT_1D2/1, AEMS_LUT_1D3/1
  Sum4/1 -> A_pade_2nd_order_filter_1/3(Vxx_b2_1)
  Constant1/1 -> Sum1/1
  Sum1/1 -> Sum2/1
  Sum2/1 -> Sum3/1
  Sum3/1 -> Sum4/1
  Saturation/1 -> Vxx_dly_1/1

== system AEMS_Standard_Library/SPECIFIC/AEMS_AS_PADE/A_pade_model/A_filter_pade/B_filter_2 ==
  Vxx_dly_t : Inport
  Vxx_dly_1 : Inport  Port=2
  Vbx_dly_init_ena : Inport  Port=3
  Vxx_in_fil : Inport  Port=4
  AEMS_LUT_1D : AEMS_Standard_Library/LOOKUP_TABLES/AEMS_LUT_1D  Tag=[LIB]  map_x=Cxb_lb_dly_t_para  map_z=Cxp_lb_b0_2
      settings: AttributesFormatString=%<MaskType>\nBkPX=%<map_x>\nLUT=%<map_z>
  AEMS_LUT_1D1 : AEMS_Standard_Library/LOOKUP_TABLES/AEMS_LUT_1D  Tag=[LIB]  map_x=Cxb_lb_dly_t_para  map_z=Cxp_lb_b1_2
      settings: AttributesFormatString=%<MaskType>\nBkPX=%<map_x>\nLUT=%<map_z>
  AEMS_LUT_1D2 : AEMS_Standard_Library/LOOKUP_TABLES/AEMS_LUT_1D  Tag=[LIB]  map_x=Cxb_lb_dly_t_para  map_z=Cxp_lb_a1_2
      settings: AttributesFormatString=%<MaskType>\nBkPX=%<map_x>\nLUT=%<map_z>
  AEMS_LUT_1D3 : AEMS_Standard_Library/LOOKUP_TABLES/AEMS_LUT_1D  Tag=[LIB]  map_x=Cxb_lb_dly_t_para  map_z=Cxp_lb_a2_2
      settings: AttributesFormatString=%<MaskType>\nBkPX=%<map_x>\nLUT=%<map_z>
  A_pade_2nd_order_filter_2 : Subsystem
  Constant1 : Constant  OutDataTypeStr=Inherit: Inherit via back propagation
  Saturation : Saturate  UpperLimit=2000  LowerLimit=0  RndMeth=Zero
      settings: AttributesFormatString=<limits=%<UpperLimit>/%<LowerLimit>>
  Sum1 : Sum  OutDataTypeStr=Inherit: Inherit via back propagation  RndMeth=Zero  InputSameDT=on
  Sum2 : Sum  OutDataTypeStr=Inherit: Inherit via back propagation  RndMeth=Zero  InputSameDT=on
  Sum3 : Sum  Inputs=+-  OutDataTypeStr=Inherit: Inherit via back propagation  RndMeth=Zero  InputSameDT=on
  Sum4 : Sum  Inputs=+-  OutDataTypeStr=Inherit: Inherit via back propagation  RndMeth=Zero  InputSameDT=on
  Vxx_dly_2 : Outport
  wires:
  Vxx_in_fil/1 -> A_pade_2nd_order_filter_2/8(Vxx_in_fil)
  Vbx_dly_init_ena/1 -> A_pade_2nd_order_filter_2/7(Vbx_dly_init_ena)
  Vxx_dly_t/1 -> AEMS_LUT_1D/1, AEMS_LUT_1D1/1, AEMS_LUT_1D2/1, AEMS_LUT_1D3/1
  Vxx_dly_1/1 -> A_pade_2nd_order_filter_2/6(Vxx_dly_1)
  A_pade_2nd_order_filter_2/1(Vxx_dly_2) -> Saturation/1
  AEMS_LUT_1D/1 -> A_pade_2nd_order_filter_2/1(Vxx_b0_2), Sum4/2
  AEMS_LUT_1D1/1 -> A_pade_2nd_order_filter_2/2(Vxx_b1_2), Sum3/2
  AEMS_LUT_1D2/1 -> A_pade_2nd_order_filter_2/4(Vxx_a1_2), Sum1/2
  AEMS_LUT_1D3/1 -> A_pade_2nd_order_filter_2/5(Vxx_a2_2), Sum2/2
  Sum4/1 -> A_pade_2nd_order_filter_2/3(Vxx_b2_2)
  Constant1/1 -> Sum1/1
  Sum1/1 -> Sum2/1
  Sum2/1 -> Sum3/1
  Sum3/1 -> Sum4/1
  Saturation/1 -> Vxx_dly_2/1

== system AEMS_Standard_Library/SPECIFIC/AEMS_AS_PADE/A_pade_model/A_filter_pade/C_filter_3 ==
  Vxx_dly_t : Inport
  Vxx_dly_2 : Inport  Port=2
  Vbx_dly_init_ena : Inport  Port=3
  Vxx_in_fil : Inport  Port=4
  AEMS_LUT_1D : AEMS_Standard_Library/LOOKUP_TABLES/AEMS_LUT_1D  Tag=[LIB]  map_x=Cxb_lb_dly_t_para  map_z=Cxp_lb_b0_3
      settings: AttributesFormatString=%<MaskType>\nBkPX=%<map_x>\nLUT=%<map_z>
  AEMS_LUT_1D1 : AEMS_Standard_Library/LOOKUP_TABLES/AEMS_LUT_1D  Tag=[LIB]  map_x=Cxb_lb_dly_t_para  map_z=Cxp_lb_b1_3
      settings: AttributesFormatString=%<MaskType>\nBkPX=%<map_x>\nLUT=%<map_z>
  AEMS_LUT_1D2 : AEMS_Standard_Library/LOOKUP_TABLES/AEMS_LUT_1D  Tag=[LIB]  map_x=Cxb_lb_dly_t_para  map_z=Cxp_lb_a1_3
      settings: AttributesFormatString=%<MaskType>\nBkPX=%<map_x>\nLUT=%<map_z>
  AEMS_LUT_1D3 : AEMS_Standard_Library/LOOKUP_TABLES/AEMS_LUT_1D  Tag=[LIB]  map_x=Cxb_lb_dly_t_para  map_z=Cxp_lb_a2_3
      settings: AttributesFormatString=%<MaskType>\nBkPX=%<map_x>\nLUT=%<map_z>
  A_pade_2nd_order_filter_3 : Subsystem
  Constant1 : Constant  OutDataTypeStr=Inherit: Inherit via back propagation
  Saturation : Saturate  UpperLimit=2000  LowerLimit=0  RndMeth=Zero
      settings: AttributesFormatString=<limits=%<UpperLimit>/%<LowerLimit>>
  Sum1 : Sum  OutDataTypeStr=Inherit: Inherit via back propagation  RndMeth=Zero  InputSameDT=on
  Sum2 : Sum  OutDataTypeStr=Inherit: Inherit via back propagation  RndMeth=Zero  InputSameDT=on
  Sum3 : Sum  Inputs=+-  OutDataTypeStr=Inherit: Inherit via back propagation  RndMeth=Zero  InputSameDT=on
  Sum4 : Sum  Inputs=+-  OutDataTypeStr=Inherit: Inherit via back propagation  RndMeth=Zero  InputSameDT=on
  Vxx_in_dly : Outport
  wires:
  Vxx_in_fil/1 -> A_pade_2nd_order_filter_3/8(Vxx_in_fil)
  AEMS_LUT_1D3/1 -> A_pade_2nd_order_filter_3/5(Vxx_a2_3), Sum2/2
  AEMS_LUT_1D2/1 -> A_pade_2nd_order_filter_3/4(Vxx_a1_3), Sum1/2
  AEMS_LUT_1D1/1 -> A_pade_2nd_order_filter_3/2(Vxx_b1_3), Sum3/2
  AEMS_LUT_1D/1 -> A_pade_2nd_order_filter_3/1(Vxx_b0_3), Sum4/2
  Vbx_dly_init_ena/1 -> A_pade_2nd_order_filter_3/7(Vbx_dly_init_ena)
  A_pade_2nd_order_filter_3/1(Vxx_in_dly) -> Saturation/1
  Vxx_dly_2/1 -> A_pade_2nd_order_filter_3/6(Vxx_dly_2)
  Vxx_dly_t/1 -> AEMS_LUT_1D/1, AEMS_LUT_1D1/1, AEMS_LUT_1D2/1, AEMS_LUT_1D3/1
  Sum4/1 -> A_pade_2nd_order_filter_3/3(Vxx_b2_3)
  Constant1/1 -> Sum1/1
  Sum1/1 -> Sum2/1
  Sum2/1 -> Sum3/1
  Sum3/1 -> Sum4/1
  Saturation/1 -> Vxx_in_dly/1

== system AEMS_Standard_Library/SPECIFIC/AEMS_AT_EHR/A_Enabled_Calculation/B_Temp_calculation_in_brick/A_Entropy_calculation ==
  Vxx_ehr_spc_cata_temp_cpy : Inport
  Vxx_ehr_sys_egaf : Inport  Port=2
  Vxx_ehr_spc_ex_gas_temp_cpy : Inport  Port=3
  Vxx_ehr_wht : Inport  Port=4
  Vxx_ehr_ext_cnvt_entr : Inport  Port=5
  Vxx_ehr_samp_t : Inport  Port=6
  Constant1 : Constant  OutDataTypeStr=Inherit: Inherit via back propagation
  Constant2 : Constant  Value=0  OutDataTypeStr=Inherit: Inherit via back propagation
  Constant3 : Constant  Value=0  OutDataTypeStr=Inherit: Inherit via back propagation
  DivisionByZero : Subsystem
  DivisionByZero1 : Subsystem
  DivisionByZero2 : Subsystem
  Product1 : Product  OutDataTypeStr=Inherit: Inherit via back propagation  RndMeth=Zero
  Product2 : Product  OutDataTypeStr=Inherit: Inherit via back propagation  RndMeth=Zero
  Product4 : Product  OutDataTypeStr=Inherit: Inherit via back propagation  RndMeth=Zero
  Saturation : Saturate  UpperLimit=6535.5  LowerLimit=0  RndMeth=Zero
      settings: AttributesFormatString=<limits=%<UpperLimit>/%<LowerLimit>>
  Saturation1 : Saturate  UpperLimit=655.35  LowerLimit=0  RndMeth=Zero
      settings: AttributesFormatString=<limits=%<UpperLimit>/%<LowerLimit>>
  Sum : Sum  Inputs=2  OutDataTypeStr=Inherit: Inherit via back propagation  RndMeth=Zero  InputSameDT=on
  Sum1 : Sum  Inputs=2  OutDataTypeStr=Inherit: Inherit via back propagation  RndMeth=Zero  InputSameDT=on
  Vxx_ehr_entr_tot : Outport
  Vxx_ehr_wht_entr : Outport  Port=2
  Vxx_ehr_ex_gas_entr : Outport  Port=3
  Vxx_ehr_wht_entr_rat : Outport  Port=4
  Vxx_ehr_ex_gas_entr_rat : Outport  Port=5
  Vxx_ehr_ext_cnvt_entr_rat : Outport  Port=6
  wires:
  Saturation1/1 -> DivisionByZero1/2(num), Vxx_ehr_ex_gas_entr/1, Sum/2
  Saturation/1 -> Vxx_ehr_wht_entr/1, DivisionByZero/2(num), Sum1/1
  Sum1/1 -> Sum/1
  Product1/1 -> Product4/1
  Sum/1 -> DivisionByZero/1(Vxx_ehr_entr_tot), DivisionByZero1/1(Vxx_ehr_entr_tot), Vxx_ehr_entr_tot/1, DivisionByZero2/1(Vxx_ehr_entr_tot)  "Vxx_ehr_entr_tot"
  Product4/1 -> Saturation1/1  "Vxx_ehr_ex_gas_entr"
  Product2/1 -> Saturation/1  "Vxx_ehr_wht_entr"
  Vxx_ehr_spc_cata_temp_cpy/1 -> Product2/1
  Vxx_ehr_spc_ex_gas_temp_cpy/1 -> Product4/2
  Vxx_ehr_wht/1 -> Product2/2
  Vxx_ehr_sys_egaf/1 -> Product1/1
  Vxx_ehr_samp_t/1 -> Product1/2
  Constant1/1 -> DivisionByZero/3(ans_of_0div)
  DivisionByZero/1(Vxx_ehr_wht_entr_rat) -> Vxx_ehr_wht_entr_rat/1
  Constant2/1 -> DivisionByZero1/3(ans_of_0div)
  DivisionByZero1/1(Vxx_ehr_ex_gas_entr_rat) -> Vxx_ehr_ex_gas_entr_rat/1
  Vxx_ehr_ext_cnvt_entr/1 -> Sum1/2, DivisionByZero2/2(num)
  Constant3/1 -> DivisionByZero2/3(ans_of_0div)
  DivisionByZero2/1(Vxx_ehr_ext_cnvt_entr_rat) -> Vxx_ehr_ext_cnvt_entr_rat/1

== system AEMS_Standard_Library/SPECIFIC/AEMS_AT_EHR/A_Enabled_Calculation/B_Temp_calculation_in_brick/B_Temp_fluctuation_calculation ==
  Vxx_ehr_entr_tot : Inport
  Vxx_ehr_wht_entr_rat : Inport  Port=2
  Vxx_ehr_ex_gas_entr_rat : Inport  Port=3
  Vxx_ehr_ext_cnvt_entr_rat : Inport  Port=4
  Vxx_ehr_samp_t : Inport  Port=5
  Vxx_ehr_exo_pow : Inport  Port=6
  Vxx_ehr_utp : Inport  Port=7
  Vxx_ehr_cata_temp_dly : Inport  Port=8
  Vxx_ehr_sel_tenv : Inport  Port=9
  Constant1 : Constant  Value=0  OutDataTypeStr=Inherit: Inherit via back propagation
  DivisionByZero : Subsystem
  Product1 : Product  Inputs=**  OutDataTypeStr=Inherit: Inherit via back propagation  RndMeth=Zero
  Product2 : Product  OutDataTypeStr=Inherit: Inherit via back propagation  RndMeth=Zero
  Product3 : Product  OutDataTypeStr=Inherit: Inherit via back propagation  RndMeth=Zero
  Product6 : Product  OutDataTypeStr=Inherit: Inherit via back propagation  RndMeth=Zero
  Vxx_ehr_exo_temp_flu : Outport
  Vxx_ehr_wht_temp_flu : Outport  Port=2
  Vxx_ehr_ex_gas_temp_flu : Outport  Port=3
  Vxx_ehr_ext_cnvt_temp_flu : Outport  Port=4
  wires:
  Constant1/1 -> DivisionByZero/3(ans_of_0div)
  DivisionByZero/1(Vxx_ehr_exo_temp_flu) -> Vxx_ehr_exo_temp_flu/1
  Product1/1 -> DivisionByZero/2(num)
  Vxx_ehr_entr_tot/1 -> DivisionByZero/1(Vxx_ehr_entr_tot)
  Vxx_ehr_exo_pow/1 -> Product1/1
  Vxx_ehr_ex_gas_entr_rat/1 -> Product2/2
  Product2/1 -> Vxx_ehr_ex_gas_temp_flu/1
  Product6/1 -> Vxx_ehr_wht_temp_flu/1
  Vxx_ehr_samp_t/1 -> Product1/2
  Product3/1 -> Vxx_ehr_ext_cnvt_temp_flu/1
  Vxx_ehr_utp/1 -> Product2/1
  Vxx_ehr_wht_entr_rat/1 -> Product6/2
  Vxx_ehr_cata_temp_dly/1 -> Product6/1
  Vxx_ehr_sel_tenv/1 -> Product3/1
  Vxx_ehr_ext_cnvt_entr_rat/1 -> Product3/2
